simulink model "Quad_Copter_mathematical_model_and_control"  (Simulink 8.1)
settings: Solver=ode3  StartTime=0.0  StopTime=30  FixedStep=0.02  RelTol=1e-3
values from neighbouring files (symbols this model uses):
  b = 1.24e-7    (= 1.24e-07)    [Quad_Copter_Constants.m]
  g = 9.81    [Quad_Copter_Constants.m]
  i_r = 1.28e-4    (= 0.000128)    [Quad_Copter_Constants.m]
  i_xx = i_yy    (= 0.008978)    [Quad_Copter_Constants.m]
  i_yy = 8.978e-3    (= 0.008978)    [Quad_Copter_Constants.m]
  i_zz = .01648    (= 0.01648)    [Quad_Copter_Constants.m]
  k = 9.595e-6    (= 9.595e-06)    [Quad_Copter_Constants.m]
  l = .25    (= 0.25)    [Quad_Copter_Constants.m]
  m = 1.1    [Quad_Copter_Constants.m]
undefined symbols (not defined in the file or in its folder): sigbuilder_block
libraries: simulink_extras x4, simulink x1, vrlib x1, aerolibutil x1, aerolibbdyn x1
settings Model: Creator=mohamed  LastModifiedBy=root
settings DataIOCC: SignalLoggingSaveFormat=Dataset
settings OptimizationCC: ExpressionDepthLimit=128
settings DebuggingCC: FcnCallInpInsideContextMsg=EnableAllAsError  StateNameClashWarn=none
settings GRTTargetCC: CodeReplacementLibrary=None  CombineOutputUpdateFcns=on  CPPClassGenCompliant=on  GRTInterface=off

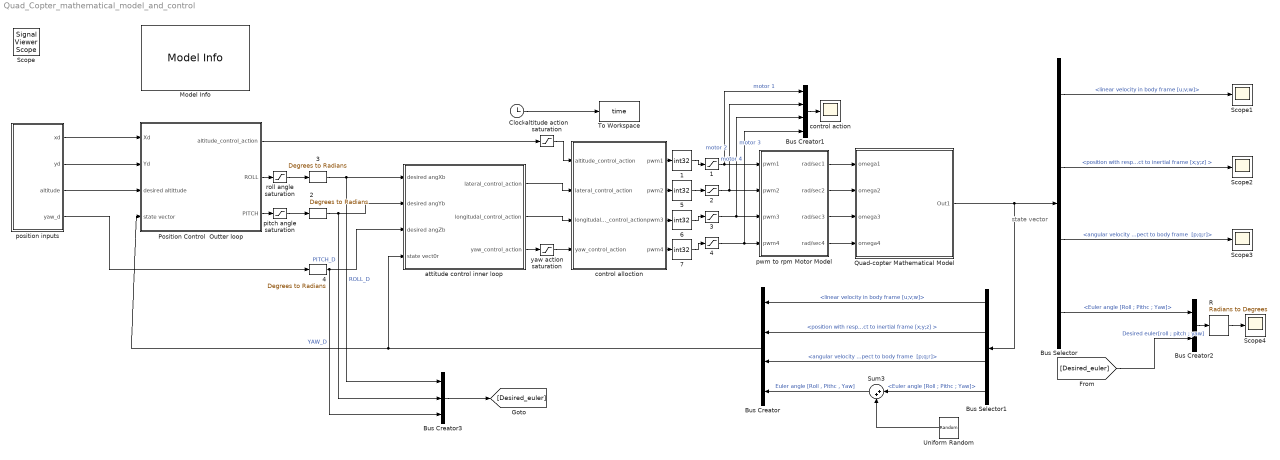
== system Quad_Copter_mathematical_model_and_control ==
  note: state vector
  " position inputs " : Subsystem  Tag=STV Subsys  LoadFcn=sigbuilder_block('load');  StartFcn=sigbuilder_block('start');  StopFcn=sigbuilder_block('stop');  ClipboardFcn=sigbuilder_block('clipboard');  mask(Sigbuilder block){}
      mask help: Simulink:masks:SigbuilderBlock_MD
      mask init:
      | if ~strcmp(get_param(bdroot(gcbh),'SimulationStatus'),'stopped') tuvar = sigbuilder_block('maskInit'); end
      settings: CopyFcn=sigbuilder_block('copy');  DeleteFcn=sigbuilder_block('delete');  ModelCloseFcn=sigbuilder_block('modelClose');  PreSaveFcn=sigbuilder_block('preSave');  PauseFcn=sigbuilder_block('pause');  ContinueFcn=sigbuilder_block('continue');  NameChangeFcn=sigbuilder_block('namechange');  OpenFcn=sigbuilder_block('open',[0.8 63.2 976.8 450.4 ]);  CloseFcn=sigbuilder_block('close');
      mask Display: plot(0, 0, 100, 100,[2, 2, 32, 32, 2], [68, 8, 8, 68, 68],[32, 2], [38, 38], [32, 19, 2],[53, 60, 44], [32, 17, 17, 2],[16, 16, 31, 31]);txt = getActiveGroup(gcbh);text(2, 100, txt,'verticalAlignment', 'top');
  {1,5..7} (4 alike) : DataTypeConversion  OutDataTypeStr=int32
  "1 " : Saturate  UpperLimit=1000  LowerLimit=0
  2 : simulink_extras/Transformations/Degrees to Radians
  "2 " : Saturate  UpperLimit=1000  LowerLimit=0
  3 : simulink_extras/Transformations/Degrees to Radians
  "3 " : Saturate  UpperLimit=1000  LowerLimit=0
  4 : simulink_extras/Transformations/Degrees to Radians
  "4 " : Saturate  UpperLimit=1000  LowerLimit=0
  Bus Creator : BusCreator
  Bus Creator1 : BusCreator
  Bus Creator2 : BusCreator  Inputs=2
  Bus Creator3 : BusCreator  Inputs=3
  Bus Selector : BusSelector  OutputSignals="linear velocity in body frame [u;v;w],position with respect to inertial frame [x;y;z] ,angular velocity with respect to body frame  [p;q;r],Euler angle [Roll ; Pithc ; Yaw]"
  Bus Selector1 : BusSelector  OutputSignals="linear velocity in body frame [u;v;w],position with respect to inertial frame [x;y;z] ,angular velocity with respect to body frame  [p;q;r],Euler angle [Roll ; Pithc ; Yaw]"
  Clock : Clock
  Model Info : simulink/Model-Wide Utilities/Model Info  InitialBlockCM=none  BlockCM=None  Frame=on  DisplayStringWithTags=|  HorizontalTextAlignment=Center  LeftAlignmentValue=0.5  SourceBlockDiagram=Quad_Copter_mathematical_model_and_control  TagMaxNumber=20
      | Model Info
      | %<Created>
      | %<ModelVersion>
      | Mohamed Gamal Abdelhady
      | Aerospace Dpt. Cairo Uni.
      | Quad Copter Model and Control
  "Position Control  Outter loop " : Subsystem
  Quad-copter Mathematical Model : Subsystem
  R : simulink_extras/Transformations/Radians to Degrees
  Scope{1..4} (4 alike) : Scope
      Scope1 settings: TickLabels=on  ShowLegends=on
      Scope2 settings: TickLabels=on  ShowLegends=on  TimeRange=20  YMin=-0.1  YMax=1.05
      Scope3 settings: TickLabels=on  ShowLegends=on  SaveName=ScopeData2
      Scope4 settings: TickLabels=on  ShowLegends=on  YMin=-0.005  YMax=0.095  SaveName=ScopeData3  SampleInput=on
  Sum3 : Sum  Inputs=|++
  To Workspace : ToWorkspace  VariableName=time  SampleTime=-1
  "Uniform Random " : UniformRandomNumber  Minimum=-0.005*pi/180  Maximum=0.005*pi/180  SampleTime=0.02
  altitude action saturation : Saturate  UpperLimit=300  LowerLimit=-300
  attitude control inner loop : Subsystem
  control action : Scope
      settings: ShowLegends=on  TimeRange=2.018561484918794  YMin=395.6594323873123  YMax=429.2153589315527  SaveName=ScopeData13
  control alloction : Subsystem
  pitch angle saturation : Saturate  UpperLimit=45  LowerLimit=-45
  pwm to rpm Motor Model : Subsystem
  roll angle saturation : Saturate  UpperLimit=45  LowerLimit=-45
  yaw action saturation : Saturate  UpperLimit=200  LowerLimit=-200
  Scope : SignalViewerScope  IOType=viewer  NumInputPorts=3  RefreshTime=0.035000
  wires:
  Bus Selector/3 -> Scope3/1  "<angular velocity with respect to body frame  [p;q;r]>"
  Bus Selector/1 -> Scope1/1  "<linear velocity in body frame [u;v;w]>"
  attitude control inner loop/1(lateral_control_action) -> control alloction/2(lateral_control_action)
  attitude control inner loop/2(longitudal_control_action) -> control alloction/3(longitudal_control_action)
  2/1 -> Bus Creator3/2, attitude control inner loop/2(desired angYb)  "PITCH_D"
  4/1 -> Bus Creator3/3, attitude control inner loop/3(desired angZb)  "YAW_D"
  Bus Creator1/1 -> control action/1
  "1 "/1 -> pwm to rpm Motor Model/1(pwm1), Bus Creator1/1  "motor 1"
  "2 "/1 -> pwm to rpm Motor Model/2(pwm2), Bus Creator1/2  "motor 2"
  "3 "/1 -> pwm to rpm Motor Model/3(pwm3), Bus Creator1/3  "motor 3"
  "4 "/1 -> pwm to rpm Motor Model/4(pwm4), Bus Creator1/4  "motor 4"
  Clock/1 -> To Workspace/1
  Bus Selector/4 -> Bus Creator2/1  "<Euler angle [Roll ; Pithc ; Yaw]>"
  pwm to rpm Motor Model/1(rad/sec1) -> Quad-copter Mathematical Model/1(omega1)
  pwm to rpm Motor Model/2(rad/sec2) -> Quad-copter Mathematical Model/2(omega2)
  pwm to rpm Motor Model/3(rad/sec3) -> Quad-copter Mathematical Model/3(omega3)
  pwm to rpm Motor Model/4(rad/sec4) -> Quad-copter Mathematical Model/4(omega4)
  " position inputs "/4(yaw_d) -> 4/1
  "Position Control  Outter loop "/3("PITCH ") -> pitch angle saturation/1
  "Position Control  Outter loop "/2(ROLL) -> roll angle saturation/1
  pitch angle saturation/1 -> 2/1
  roll angle saturation/1 -> 3/1
  Bus Selector/2 -> Scope2/1  "<position with respect to inertial frame [x;y;z] >"
  " position inputs "/2(yd) -> "Position Control  Outter loop "/2(Yd)
  " position inputs "/1(xd) -> "Position Control  Outter loop "/1(Xd)
  " position inputs "/3(altitude) -> "Position Control  Outter loop "/3(desired altittude)
  "Position Control  Outter loop "/1(altitude_control_action) -> altitude action saturation/1
  attitude control inner loop/3(yaw_control_action) -> yaw action saturation/1
  Quad-copter Mathematical Model/1(Out1) -> Bus Selector1/1, Bus Selector/1
  Bus Selector1/2 -> Bus Creator/2  "<position with respect to inertial frame [x;y;z] >"
  Bus Selector1/1 -> Bus Creator/1  "<linear velocity in body frame [u;v;w]>"
  Bus Selector1/3 -> Bus Creator/3  "<angular velocity with respect to body frame  [p;q;r]>"
  Bus Creator/1 -> attitude control inner loop/4(state vect0r), "Position Control  Outter loop "/4(state vector)
  "Uniform Random "/1 -> Sum3/2
  Bus Selector1/4 -> Sum3/1  "<Euler angle [Roll ; Pithc ; Yaw]>"
  Sum3/1 -> Bus Creator/4  "Euler angle [Roll , Pithc , Yaw]"
  control alloction/1(pwm1) -> 1/1
  1/1 -> "1 "/1
  control alloction/2(pwm2) -> 5/1
  control alloction/3(pwm3) -> 6/1
  control alloction/4(pwm4) -> 7/1
  5/1 -> "2 "/1
  6/1 -> "3 "/1
  7/1 -> "4 "/1
  3/1 -> Bus Creator3/1, attitude control inner loop/1(desired angXb)  "ROLL_D"
  Bus Creator3/1 -> [Desired_euler]
  [Desired_euler] -> Bus Creator2/2  "Desired euler[roll ; pitch ; yaw]"
  Bus Creator2/1 -> R/1
  R/1 -> Scope4/1
  yaw action saturation/1 -> control alloction/4(yaw_control_action)
  altitude action saturation/1 -> control alloction/1(altitude_control_action)

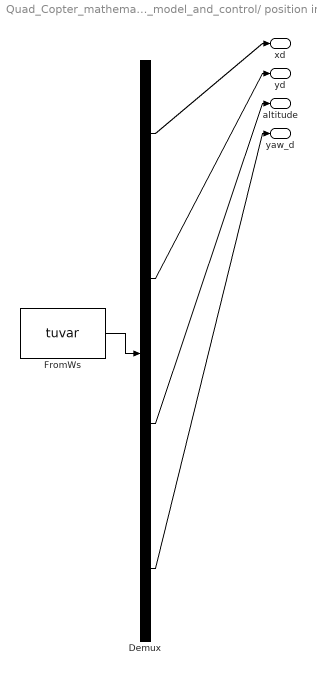
== system Quad_Copter_mathematical_model_and_control/ position inputs  ==
  Demux : Demux  Tag=STV Demux
  FromWs : FromWorkspace  Tag=STV FromWs  VariableName=tuvar  SampleTime=0  SigBuilderData=DataTag0  VnvData=DataTag1
      SigBuilderData=|
      | common.afterFinalStr = 'Extrapolate'
      | common.sampleTime = 0
      | dataSet.timeRange = [0 20]
      | dataSet.name = 'Group 1'
      | sbobj.Groups.Name = 'Group 1'
      | sbobj.Groups.Signals(1).Name = 'xd'
      | sbobj.Groups.Signals(1).XData = [0 2.04 2.04 20]
      | sbobj.Groups.Signals(1).YData = [0 0 3 3]
      | sbobj.Groups.Signals(2).Name = 'yd'
      | sbobj.Groups.Signals(2).XData = [0 15.92 15.92 20]
      | sbobj.Groups.Signals(2).YData = [0 0 -3 -3]
      | sbobj.Groups.Signals(3).Name = 'altitude'
      | sbobj.Groups.Signals(3).XData = [0 8 8 20]
      | sbobj.Groups.Signals(3).YData = [0 0 1 1]
      | sbobj.Groups.Signals(4).Name = 'yaw_d'
      | sbobj.Groups.Signals(4).XData = [0 20]
      | sbobj.Groups.Signals(4).YData = [0 0]
      | sbobj.Groups.TimeRange = [0 20]
  xd : Outport  Tag=STV Outport
  yd : Outport  Tag=STV Outport  Port=2
  altitude : Outport  Tag=STV Outport  Port=3
  yaw_d : Outport  Tag=STV Outport  Port=4
  wires:
  FromWs/1 -> Demux/1
  Demux/1 -> xd/1
  Demux/2 -> yd/1
  Demux/3 -> altitude/1
  Demux/4 -> yaw_d/1

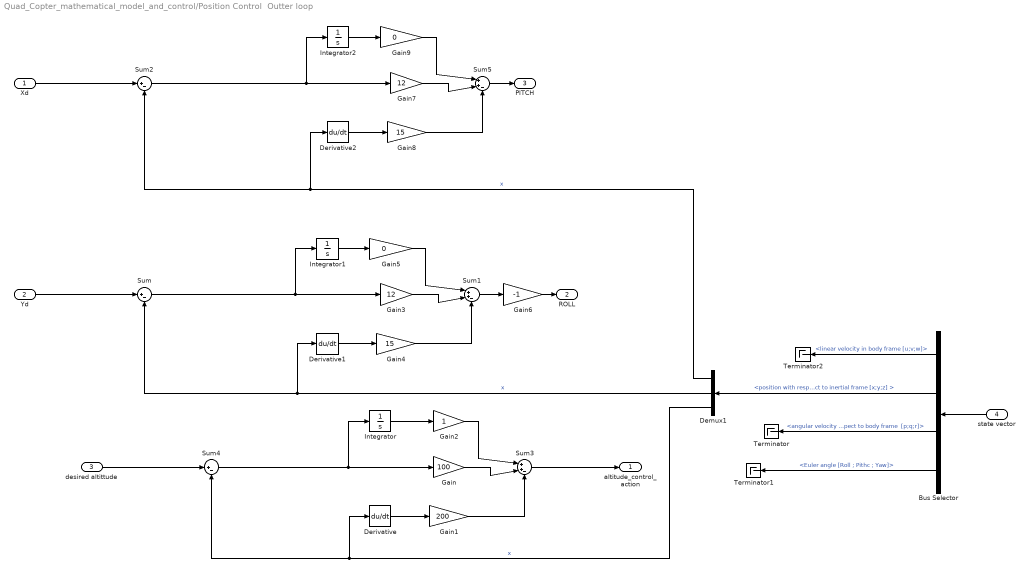
== system Quad_Copter_mathematical_model_and_control/Position Control  Outter loop  ==
  Xd : Inport
  Yd : Inport  Port=2
  desired altittude : Inport  Port=3
  state vector : Inport  Port=4
  Bus Selector : BusSelector  OutputSignals="linear velocity in body frame [u;v;w],position with respect to inertial frame [x;y;z] ,angular velocity with respect to body frame  [p;q;r],Euler angle [Roll ; Pithc ; Yaw]"
  Demux1 : Demux  Outputs=3
  Derivative : Derivative  CoefficientInTFapproximation=0.001
  Derivative1 : Derivative  CoefficientInTFapproximation=0.001
  Derivative2 : Derivative  CoefficientInTFapproximation=0.001
  Gain : Gain  Gain=100
  Gain1 : Gain  Gain=200
  Gain2 : Gain
  Gain3 : Gain  Gain=12
  Gain4 : Gain  Gain=15
  Gain5 : Gain  Gain=0
  Gain6 : Gain  Gain=-1
  Gain7 : Gain  Gain=12
  Gain8 : Gain  Gain=15
  Gain9 : Gain  Gain=0
  Integrator : Integrator
  Integrator1 : Integrator
  Integrator2 : Integrator
  Sum : Sum  Inputs=|+-
  Sum1 : Sum  Inputs=|++-
  Sum2 : Sum  Inputs=|+-
  Sum3 : Sum  Inputs=|++-
  Sum4 : Sum  Inputs=|+-
  Sum5 : Sum  Inputs=|++-
  Terminator : Terminator
  Terminator1 : Terminator
  Terminator2 : Terminator
  altitude_control_action : Outport
  ROLL : Outport  Port=2
  "PITCH " : Outport  Port=3
  wires:
  Yd/1 -> Sum/1
  Xd/1 -> Sum2/1
  Bus Selector/3 -> Terminator/1  "<angular velocity with respect to body frame  [p;q;r]>"
  Bus Selector/2 -> Demux1/1  "<position with respect to inertial frame [x;y;z] >"
  Bus Selector/1 -> Terminator2/1  "<linear velocity in body frame [u;v;w]>"
  state vector/1 -> Bus Selector/1
  desired altittude/1 -> Sum4/1
  Gain6/1 -> ROLL/1
  Demux1/2 -> Derivative1/1, Sum/2  "x"
  Gain3/1 -> Sum1/2
  Derivative1/1 -> Gain4/1
  Gain4/1 -> Sum1/3
  Sum/1 -> Integrator1/1, Gain3/1
  Integrator1/1 -> Gain5/1
  Gain5/1 -> Sum1/1
  Sum1/1 -> Gain6/1
  Bus Selector/4 -> Terminator1/1  "<Euler angle [Roll ; Pithc ; Yaw]>"
  Demux1/1 -> Derivative2/1, Sum2/2  "x"
  Gain7/1 -> Sum5/2
  Derivative2/1 -> Gain8/1
  Gain8/1 -> Sum5/3
  Sum2/1 -> Integrator2/1, Gain7/1
  Integrator2/1 -> Gain9/1
  Gain9/1 -> Sum5/1
  Sum5/1 -> "PITCH "/1
  Demux1/3 -> Derivative/1, Sum4/2  "x"
  Gain/1 -> Sum3/2
  Derivative/1 -> Gain1/1
  Gain1/1 -> Sum3/3
  Sum4/1 -> Gain/1, Integrator/1
  Integrator/1 -> Gain2/1
  Gain2/1 -> Sum3/1
  Sum3/1 -> altitude_control_action/1

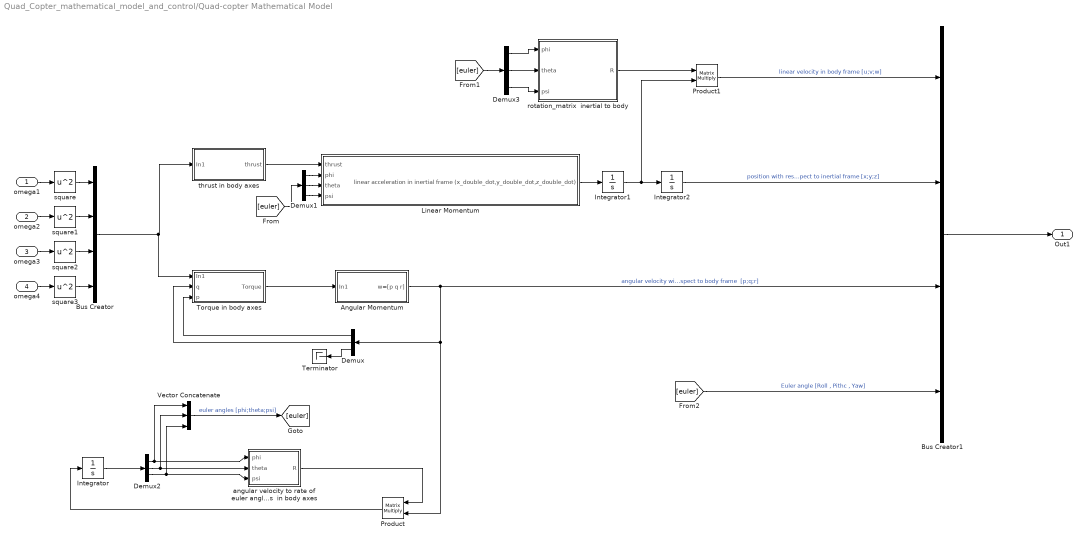
== system Quad_Copter_mathematical_model_and_control/Quad-copter Mathematical Model ==
  omega1 : Inport
  omega2 : Inport  Port=2
  omega3 : Inport  Port=3
  omega4 : Inport  Port=4
  Angular Momentum : Subsystem
  Bus Creator : BusCreator
  Bus Creator1 : BusCreator
  Demux{,1..3} (4 alike) : Demux  Outputs=3
  Integrator : Integrator
  Integrator1 : Integrator
  Integrator2 : Integrator
  Linear Momentum : Subsystem
  Product : Product  Inputs=**  Multiplication=Matrix(*)
  Product1 : Product  Inputs=**  Multiplication=Matrix(*)
  Terminator : Terminator
  Torque in body axes : Subsystem
  Vector Concatenate : Concatenate  NumInputs=3
  angular velocity to rate of euler angles  in body axes : MATLAB Function  TreatAsAtomicUnit=on
  rotation_matrix  inertial to body : MATLAB Function  TreatAsAtomicUnit=on
  square{,1..3} (4 alike) : Math  Operator=square  SaturateOnIntegerOverflow=on
  thrust in body axes : Subsystem
  Out1 : Outport
  wires:
  omega1/1 -> square/1
  omega2/1 -> square1/1
  omega3/1 -> square2/1
  omega4/1 -> square3/1
  Bus Creator/1 -> Torque in body axes/1(In1), thrust in body axes/1(In1)
  Torque in body axes/1(Torque) -> Angular Momentum/1(In1)
  thrust in body axes/1(thrust) -> Linear Momentum/1(thrust)
  Angular Momentum/1(w=[p q r]) -> Product/2, Demux/1, Bus Creator1/3  "angular velocity with respect to body frame  [p;q;r]"
  square/1 -> Bus Creator/1
  square1/1 -> Bus Creator/2
  square2/1 -> Bus Creator/3
  square3/1 -> Bus Creator/4
  Demux/3 -> Terminator/1
  Linear Momentum/1(linear acceleration in inertial frame (x_double_dot,y_double_dot,z_double_dot)) -> Integrator1/1
  Product/1 -> Integrator/1
  Integrator/1 -> Demux2/1
  Demux2/1 -> angular velocity to rate of euler angles  in body axes/1(phi), Vector Concatenate/1
  Demux2/2 -> angular velocity to rate of euler angles  in body axes/2(theta), Vector Concatenate/2
  Demux2/3 -> angular velocity to rate of euler angles  in body axes/3(psi), Vector Concatenate/3
  angular velocity to rate of euler angles  in body axes/1(R) -> Product/1
  Vector Concatenate/1 -> [euler]  "euler angles [phi;theta;psi]"
  Integrator1/1 -> Product1/2, Integrator2/1
  Integrator2/1 -> Bus Creator1/2  "position with respect to inertial frame [x;y;z]"
  [euler] -> Demux1/1
  Demux1/2 -> Linear Momentum/3(theta)
  Demux1/1 -> Linear Momentum/2(phi)
  Demux1/3 -> Linear Momentum/4(psi)
  [euler] -> Demux3/1
  Demux3/3 -> rotation_matrix  inertial to body/3(psi)
  Demux3/2 -> rotation_matrix  inertial to body/2(theta)
  Demux3/1 -> rotation_matrix  inertial to body/1(phi)
  rotation_matrix  inertial to body/1(R) -> Product1/1
  Product1/1 -> Bus Creator1/1  "linear velocity in body frame [u;v;w]"
  Bus Creator1/1 -> Out1/1
  Demux/1 -> Torque in body axes/3(p)
  Demux/2 -> Torque in body axes/2(q)
  [euler] -> Bus Creator1/4  "Euler angle [Roll , Pithc , Yaw]"

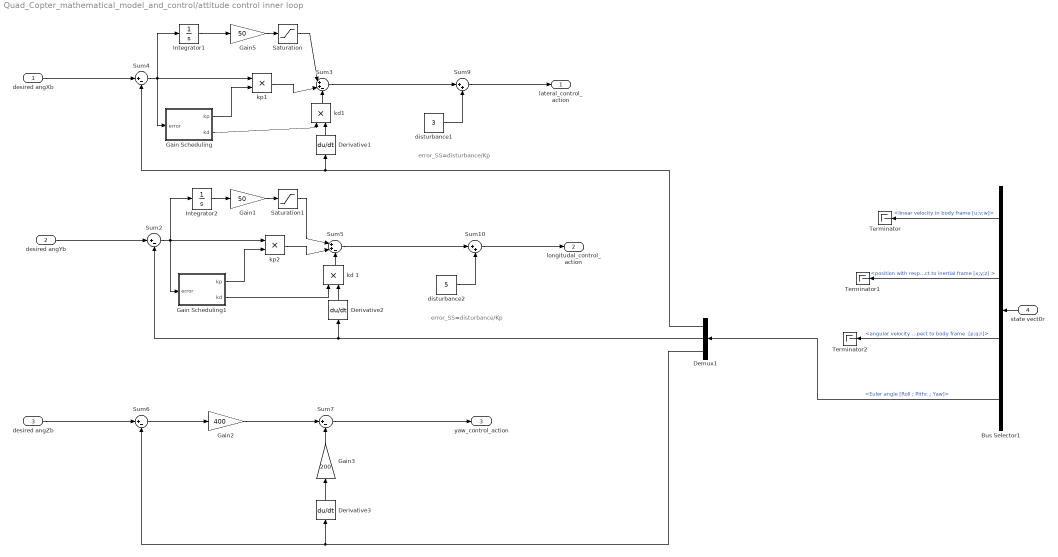
== system Quad_Copter_mathematical_model_and_control/attitude control inner loop ==
  note: error_SS=disturbance/Kp
  note: error_SS=disturbance/Kp
  desired angXb : Inport
  desired angYb : Inport  Port=2
  desired angZb : Inport  Port=3
  state vect0r : Inport  Port=4
  Bus Selector1 : BusSelector  OutputSignals="linear velocity in body frame [u;v;w],position with respect to inertial frame [x;y;z] ,angular velocity with respect to body frame  [p;q;r],Euler angle [Roll ; Pithc ; Yaw]"
  Demux1 : Demux  Outputs=3
  Derivative1 : Derivative  CoefficientInTFapproximation=0.001
  Derivative2 : Derivative  CoefficientInTFapproximation=0.001
  Derivative3 : Derivative  CoefficientInTFapproximation=0.001
  Gain Scheduling : MATLAB Function  TreatAsAtomicUnit=on
  Gain Scheduling1 : MATLAB Function  TreatAsAtomicUnit=on
  Gain1 : Gain  Gain=50
  Gain2 : Gain  Gain=400
  Gain3 : Gain  Gain=200
  Gain5 : Gain  Gain=50
  Integrator1 : Integrator  LimitOutput=on  UpperSaturationLimit=100/50  LowerSaturationLimit=-100/50
  Integrator2 : Integrator  LimitOutput=on  UpperSaturationLimit=100/50  LowerSaturationLimit=-100/50
  Saturation : Saturate  UpperLimit=100  LowerLimit=-100
  Saturation1 : Saturate  UpperLimit=100  LowerLimit=-100
  Sum10 : Sum  Inputs=|++
  Sum{2,4,6..7} (4 alike) : Sum  Inputs=|+-
  Sum3 : Sum  Inputs=|++-
  Sum5 : Sum  Inputs=|++-
  Sum9 : Sum  Inputs=|++
  Terminator : Terminator
  Terminator1 : Terminator
  Terminator2 : Terminator
  disturbance1 : Constant  Value=3
  disturbance2 : Constant  Value=5
  kd 1 : Product  Inputs=**
  "kd1 " : Product  Inputs=**
  kp1 : Product  Inputs=**
  kp2 : Product  Inputs=**
  lateral_control_action : Outport
  longitudal_control_action : Outport  Port=2
  yaw_control_action : Outport  Port=3
  wires:
  desired angYb/1 -> Sum2/1
  desired angXb/1 -> Sum4/1
  desired angZb/1 -> Sum6/1
  Demux1/3 -> Sum6/2, Derivative3/1
  disturbance1/1 -> Sum9/2
  Sum9/1 -> lateral_control_action/1
  Demux1/1 -> Derivative1/1, Sum4/2
  Sum3/1 -> Sum9/1
  Gain Scheduling/1(kp) -> kp1/2
  Derivative1/1 -> "kd1 "/2
  Gain Scheduling/2(kd) -> "kd1 "/1
  "kd1 "/1 -> Sum3/3
  kp1/1 -> Sum3/2
  disturbance2/1 -> Sum10/2
  Sum10/1 -> longitudal_control_action/1
  Demux1/2 -> Derivative2/1, Sum2/2
  Sum5/1 -> Sum10/1
  Gain Scheduling1/1(kp) -> kp2/2
  Derivative2/1 -> kd 1/2
  Gain Scheduling1/2(kd) -> kd 1/1
  kd 1/1 -> Sum5/3
  kp2/1 -> Sum5/2
  Sum4/1 -> Integrator1/1, kp1/1, Gain Scheduling/1(error)
  Integrator1/1 -> Gain5/1
  Gain5/1 -> Saturation/1
  Sum2/1 -> Gain Scheduling1/1(error), Integrator2/1, kp2/1
  Integrator2/1 -> Gain1/1
  Gain1/1 -> Saturation1/1
  Sum6/1 -> Gain2/1
  Gain2/1 -> Sum7/1
  Derivative3/1 -> Gain3/1
  Gain3/1 -> Sum7/2
  Saturation/1 -> Sum3/1
  Saturation1/1 -> Sum5/1
  Sum7/1 -> yaw_control_action/1
  state vect0r/1 -> Bus Selector1/1
  Bus Selector1/1 -> Terminator/1  "<linear velocity in body frame [u;v;w]>"
  Bus Selector1/2 -> Terminator1/1  "<position with respect to inertial frame [x;y;z] >"
  Bus Selector1/3 -> Terminator2/1  "<angular velocity with respect to body frame  [p;q;r]>"
  Bus Selector1/4 -> Demux1/1  "<Euler angle [Roll ; Pithc ; Yaw]>"

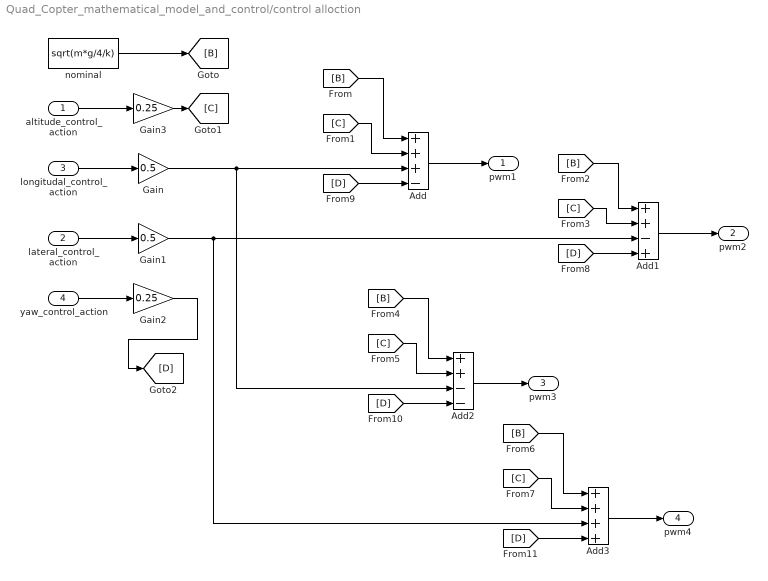
== system Quad_Copter_mathematical_model_and_control/control alloction ==
  altitude_control_action : Inport
  lateral_control_action : Inport  Port=2
  longitudal_control_action : Inport  Port=3
  yaw_control_action : Inport  Port=4
  Add : Sum  Inputs=+++-
  Add1 : Sum  Inputs=++-+
  Add2 : Sum  Inputs=++--
  Add3 : Sum  Inputs=++++
  Gain : Gain  Gain=0.5
  Gain1 : Gain  Gain=0.5
  Gain2 : Gain  Gain=0.25
  Gain3 : Gain  Gain=0.25
  nominal : Constant  Value=sqrt(m*g/4/k)
  pwm1 : Outport
  pwm2 : Outport  Port=2
  pwm3 : Outport  Port=3
  pwm4 : Outport  Port=4
  wires:
  [D] -> Add3/4
  [D] -> Add2/4
  [D] -> Add/4
  [D] -> Add1/4
  Gain2/1 -> [D]
  Gain1/1 -> Add1/3, Add3/3
  Gain/1 -> Add2/3, Add/3
  [C] -> Add3/2
  [B] -> Add3/1
  Add3/1 -> pwm4/1
  [C] -> Add2/2
  [B] -> Add2/1
  Add2/1 -> pwm3/1
  [C] -> Add1/2
  [B] -> Add1/1
  Add1/1 -> pwm2/1
  [C] -> Add/2
  Gain3/1 -> [C]
  altitude_control_action/1 -> Gain3/1
  yaw_control_action/1 -> Gain2/1
  longitudal_control_action/1 -> Gain/1
  lateral_control_action/1 -> Gain1/1
  [B] -> Add/1
  nominal/1 -> [B]
  Add/1 -> pwm1/1

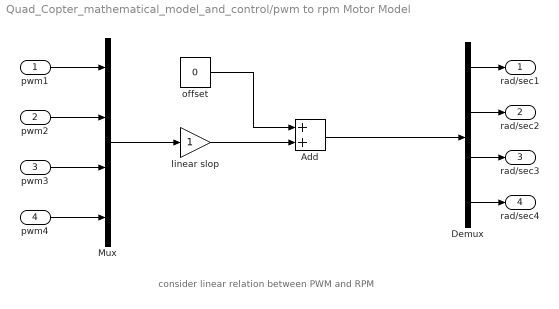
== system Quad_Copter_mathematical_model_and_control/pwm to rpm Motor Model ==
  note: consider linear relation between PWM and RPM
  pwm1 : Inport
  pwm2 : Inport  Port=2
  pwm3 : Inport  Port=3
  pwm4 : Inport  Port=4
  Add : Sum
  Demux : Demux
  Mux : Mux
  linear slop : Gain
  offset : Constant  Value=0
  rad/sec1 : Outport
  rad/sec2 : Outport  Port=2
  rad/sec3 : Outport  Port=3
  rad/sec4 : Outport  Port=4
  wires:
  pwm1/1 -> Mux/1
  pwm2/1 -> Mux/2
  pwm3/1 -> Mux/3
  pwm4/1 -> Mux/4
  Mux/1 -> linear slop/1
  linear slop/1 -> Add/2
  offset/1 -> Add/1
  Demux/1 -> rad/sec1/1
  Demux/2 -> rad/sec2/1
  Demux/3 -> rad/sec3/1
  Demux/4 -> rad/sec4/1
  Add/1 -> Demux/1

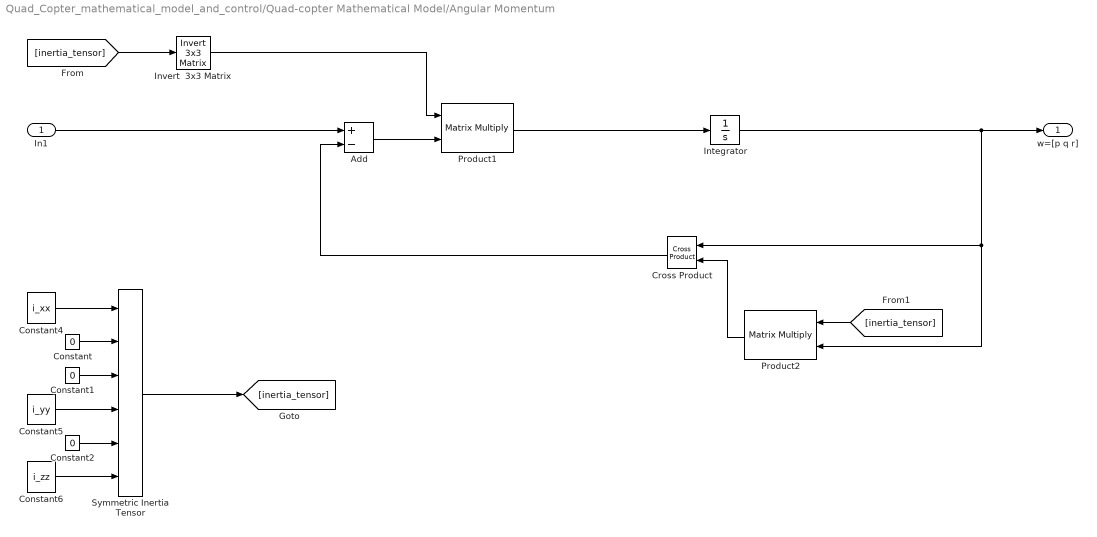
== system Quad_Copter_mathematical_model_and_control/Quad-copter Mathematical Model/Angular Momentum ==
  In1 : Inport
  Add : Sum  Inputs=+-
  Constant : Constant  Value=0
  Constant1 : Constant  Value=0
  Constant2 : Constant  Value=0
  Constant4 : Constant  Value=i_xx
  Constant5 : Constant  Value=i_yy
  Constant6 : Constant  Value=i_zz
  Cross Product : vrlib/Utilities/Cross Product
  Integrator : Integrator
  Invert  3x3 Matrix : aerolibutil/Invert  3x3 Matrix
  Product1 : Product  Inputs=**  Multiplication=Matrix(*)
  Product2 : Product  Inputs=**  Multiplication=Matrix(*)
  Symmetric Inertia Tensor : aerolibbdyn/Symmetric Inertia Tensor
  w=[p q r] : Outport
  wires:
  Product1/1 -> Integrator/1
  Constant/1 -> Symmetric Inertia Tensor/2
  Constant1/1 -> Symmetric Inertia Tensor/3
  Constant2/1 -> Symmetric Inertia Tensor/5
  Constant4/1 -> Symmetric Inertia Tensor/1
  Constant5/1 -> Symmetric Inertia Tensor/4
  Constant6/1 -> Symmetric Inertia Tensor/6
  Integrator/1 -> Product2/2, Cross Product/1, w=[p q r]/1
  In1/1 -> Add/1
  Cross Product/1 -> Add/2
  Invert  3x3 Matrix/1 -> Product1/1
  Add/1 -> Product1/2
  Product2/1 -> Cross Product/2
  Symmetric Inertia Tensor/1 -> [inertia_tensor]
  [inertia_tensor] -> Invert  3x3 Matrix/1
  [inertia_tensor] -> Product2/1

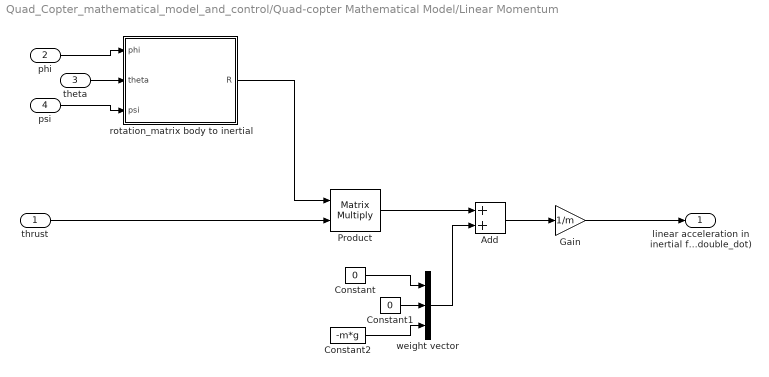
== system Quad_Copter_mathematical_model_and_control/Quad-copter Mathematical Model/Linear Momentum ==
  thrust : Inport
  phi : Inport  Port=2
  theta : Inport  Port=3
  psi : Inport  Port=4
  Add : Sum
  Constant : Constant  Value=0
  Constant1 : Constant  Value=0
  Constant2 : Constant  Value=-m*g
  Gain : Gain  Gain=1/m
  Product : Product  Multiplication=Matrix(*)
  rotation_matrix body to inertial : MATLAB Function  TreatAsAtomicUnit=on
  weight vector : Concatenate  NumInputs=3
  linear acceleration in inertial frame (x_double_dot,y_double_dot,z_double_dot) : Outport
  wires:
  rotation_matrix body to inertial/1(R) -> Product/1
  thrust/1 -> Product/2
  Product/1 -> Add/1
  Constant/1 -> weight vector/1
  Constant1/1 -> weight vector/2
  Constant2/1 -> weight vector/3
  weight vector/1 -> Add/2
  Add/1 -> Gain/1
  Gain/1 -> linear acceleration in inertial frame (x_double_dot,y_double_dot,z_double_dot)/1
  theta/1 -> rotation_matrix body to inertial/2(theta)
  phi/1 -> rotation_matrix body to inertial/1(phi)
  psi/1 -> rotation_matrix body to inertial/3(psi)

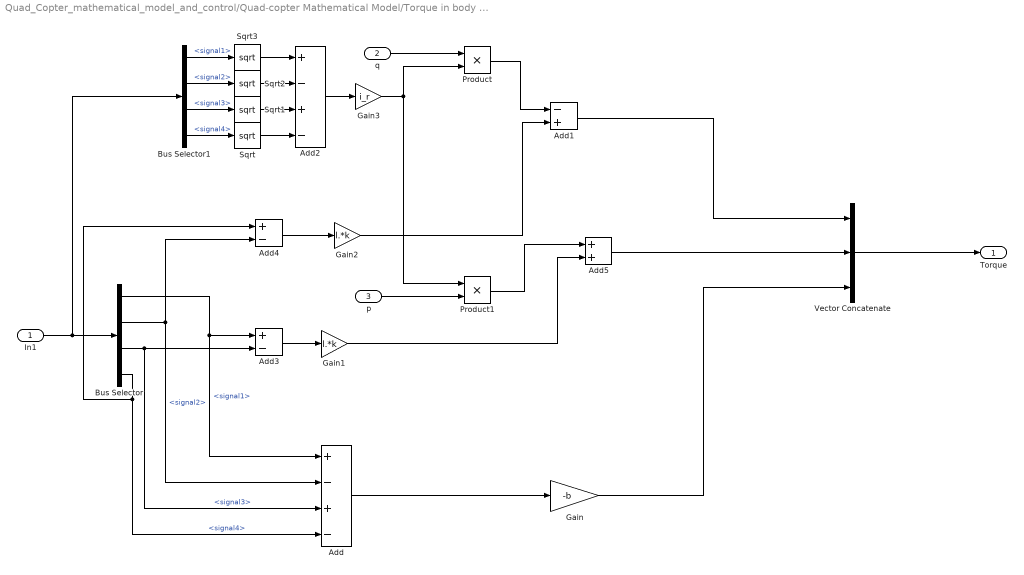
== system Quad_Copter_mathematical_model_and_control/Quad-copter Mathematical Model/Torque in body axes ==
  In1 : Inport
  q : Inport  Port=2
  p : Inport  Port=3
  Add : Sum  Inputs=+-+-
  Add1 : Sum  Inputs=-+
  Add2 : Sum  Inputs=+-+-
  Add3 : Sum  Inputs=+-
  Add4 : Sum  Inputs=+-
  Add5 : Sum
  Bus Selector : BusSelector  OutputSignals=signal1,signal2,signal3,signal4
  Bus Selector1 : BusSelector  OutputSignals=signal1,signal2,signal3,signal4
  Gain : Gain  Gain=-b
  Gain1 : Gain  Gain=l.*k
  Gain2 : Gain  Gain=l.*k
  Gain3 : Gain  Gain=i_r
  Product : Product
  Product1 : Product
  Sqrt{,1..3} (4 alike) : Sqrt  SaturateOnIntegerOverflow=on
  Vector Concatenate : Concatenate  NumInputs=3
  Torque : Outport
  wires:
  Vector Concatenate/1 -> Torque/1
  Bus Selector/1 -> Add3/1, Add/1  "<signal1>"
  Bus Selector/2 -> Add/2, Add4/2  "<signal2>"
  Bus Selector/3 -> Add3/2, Add/3  "<signal3>"
  Bus Selector/4 -> Add4/1, Add/4  "<signal4>"
  Add/1 -> Gain/1
  Add3/1 -> Gain1/1
  Add4/1 -> Gain2/1
  In1/1 -> Bus Selector1/1, Bus Selector/1
  Bus Selector1/2 -> Sqrt2/1  "<signal2>"
  Bus Selector1/3 -> Sqrt1/1  "<signal3>"
  Bus Selector1/4 -> Sqrt/1  "<signal4>"
  Bus Selector1/1 -> Sqrt3/1  "<signal1>"
  Gain2/1 -> Add1/2
  Add2/1 -> Gain3/1
  Gain3/1 -> Product/2, Product1/1
  q/1 -> Product/1
  Add1/1 -> Vector Concatenate/1
  Gain/1 -> Vector Concatenate/3
  Gain1/1 -> Add5/2
  p/1 -> Product1/2
  Add5/1 -> Vector Concatenate/2
  Sqrt/1 -> Add2/4
  Sqrt1/1 -> Add2/3
  Sqrt2/1 -> Add2/2
  Sqrt3/1 -> Add2/1
  Product/1 -> Add1/1
  Product1/1 -> Add5/1

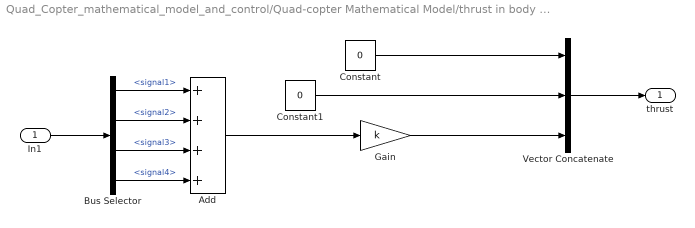
== system Quad_Copter_mathematical_model_and_control/Quad-copter Mathematical Model/thrust in body axes ==
  In1 : Inport
  Add : Sum  Inputs=++++
  Bus Selector : BusSelector  OutputSignals=signal1,signal2,signal3,signal4
  Constant : Constant  Value=0
  Constant1 : Constant  Value=0
  Gain : Gain  Gain=k
  Vector Concatenate : Concatenate  NumInputs=3
  thrust : Outport
  wires:
  In1/1 -> Bus Selector/1
  Bus Selector/1 -> Add/1  "<signal1>"
  Vector Concatenate/1 -> thrust/1
  Bus Selector/4 -> Add/4  "<signal4>"
  Bus Selector/2 -> Add/2  "<signal2>"
  Bus Selector/3 -> Add/3  "<signal3>"
  Add/1 -> Gain/1
  Gain/1 -> Vector Concatenate/3
  Constant1/1 -> Vector Concatenate/2
  Constant/1 -> Vector Concatenate/1

== matlab function Quad-copter Mathematical Model/angular velocity to rate of euler angles in body axes ==
  data: phi input double; theta input double; psi input double; R output double
function R = fcn(phi,theta,psi)
%#from angular velocity to rate of euler angles in body axes

%[phi_dot;theta_dot;psi_dot]=R*[w_x;w_y;w_z]=R*[p,q,r]
%{
algorithm
syms psi theta phi x_phi y_theta z_psi R1

z_psi=[cos(psi) -sin(psi) 0;sin(psi) cos(psi) 0;0 0 1];
y_theta=[cos(theta) 0 sin(theta);0 1 0;-sin(theta) 0 cos(theta)];
x_phi=[1 0 0;0 cos(phi) -sin(phi);0 sin(phi) cos(phi)];
identity=[1 0 0;0 1 0;0 0 1]

R1=[inv(x_phi)*inv(y_theta) inv(x_phi) identity];

R2=simplify([R1(1:3,3),R1(1:3,5),R1(1:3,7)])
R=simplify(inv(R2))
%}


R =[ 1, (sin(phi)*sin(theta))/cos(theta), (cos(phi)*sin(theta))/cos(theta);0, cos(phi),-sin(phi); 0, sin(phi)/cos(theta),cos(phi)/cos(theta)];

== matlab function Quad-copter Mathematical Model/Linear Momentum/rotation_matrix body to inertial ==
  data: phi input double; theta input double; psi input double; R output double
function R = rotation_matrix(phi,theta,psi) 
%#eulerangles about zyx(psi,thaet,phi)transform from body axes to inertial frame
z_psi=[cos(psi) -sin(psi) 0;sin(psi) cos(psi) 0;0 0 1];
y_theta=[cos(theta) 0 sin(theta);0 1 0;-sin(theta) 0 cos(theta)];
x_phi=[1 0 0;0 cos(phi) -sin(phi);0 sin(phi) cos(phi)];

R=z_psi*y_theta*x_phi;

== matlab function Quad-copter Mathematical Model/rotation_matrix inertial to body ==
  data: phi input double; theta input double; psi input double; R output double
function R = rotation_matrix(phi,theta,psi) 
%#eulerangles about zyx(psi,thaet,phi),transform from inertial frame to body frame
z_psi=[cos(psi) -sin(psi) 0;sin(psi) cos(psi) 0;0 0 1];
y_theta=[cos(theta) 0 sin(theta);0 1 0;-sin(theta) 0 cos(theta)];
x_phi=[1 0 0;0 cos(phi) -sin(phi);0 sin(phi) cos(phi)];

R=inv(z_psi*y_theta*x_phi);

== matlab function attitude control inner loop/Gain Scheduling ==
  data: error input double; kp output double; kd output double
function [kp,kd] = fcn(error)

e=abs(error);


if e<=pi/180*15
    kp=180;
    kd=70;
  
elseif e<=pi/180*25
    kp=180 - 15;
    kd=70 - 10;
elseif e<=pi/180*55
    kp=180 - 2*15;
    kd=70 - 2*10;   

else
  
    kp=180 - 3*15;
    kd=70 - 3*10;
end
    
end

== matlab function attitude control inner loop/Gain Scheduling1 ==
  data: error input double; kp output double; kd output double
function [kp,kd] = fcn(error)

e=abs(error);


if e<=pi/180*15
    kp=180;
    kd=70;
  
elseif e<=pi/180*25
    kp=180 - 15;
    kd=70 - 10;
elseif e<=pi/180*55
    kp=180 - 2*15;
    kd=70 - 2*10;   

else
  
    kp=180 - 3*15;
    kd=70 - 3*10;
end
    
end
